simulink model "DCM_Controller_Implementation_Drive2"  (R2025a)
settings: Solver=ode5  StartTime=0.0  StopTime=t_end  FixedStep=dt  RelTol=1e-3
values from neighbouring files (symbols this model uses):
  a1 = -1.122    [Experiment_2_DCM_Parameter.m]
  a2 = 2.553    [Experiment_2_DCM_Parameter.m]
  a3 = -0.759    [Experiment_2_DCM_Parameter.m]
  b1 = 0.0876    [Experiment_2_DCM_Parameter.m]
  b2 = 0.1030    (= 0.103)    [Experiment_2_DCM_Parameter.m]
  b3 = 4.8586    [Experiment_2_DCM_Parameter.m]
  C_M = 0.96    [Experiment_2_DCM_Parameter.m]
  dt = 5e-6    (= 5e-06)    [Experiment_2_DCM_Parameter.m]
  dt_omega = 5e-4    (= 0.0005)    [Experiment_2_DCM_Parameter.m]
  EncoderLines = 4096    [Experiment_2_DCM_Parameter.m]
  I_AN = 1    [Experiment_2_DCM_Parameter.m]
  I_EN = 0.1    [Experiment_2_DCM_Parameter.m]
  K_i_i = V_r_I_A/T_n_I_A    (= 16.6666666667)    [Experiment_2_DCM_Parameter.m]
  K_i_omega = V_r_omega_m/T_n_omega_m    (= 4.70196759259)    [Experiment_2_DCM_Parameter.m]
  K_p_i = V_r_I_A    (= 0.283333333333)    [Experiment_2_DCM_Parameter.m]
  K_p_omega = V_r_omega_m    (= 0.112847222222)    [Experiment_2_DCM_Parameter.m]
  n_Igain = 0.075    [Experiment_2_DCM_Parameter.m]
  n_Imax = 0.15    [Experiment_2_DCM_Parameter.m]
  n_Imin = -n_Imax    (= -0.15)    [Experiment_2_DCM_Parameter.m]
  Omega_MN = N_N*pi/30    (= 209.439510239)    [Experiment_2_DCM_Parameter.m]
  Psi_EN = 1    [Experiment_2_DCM_Parameter.m]
  R_A = 22    [Experiment_2_DCM_Parameter.m]
  R_E = 2200    [Experiment_2_DCM_Parameter.m]
  T_A = L_A/R_A    (= 0.017)    [Experiment_2_DCM_Parameter.m]
  T_c = 1/1000    (= 0.001)    [Experiment_2_DCM_Parameter.m]
  T_CON = T_c    (= 0.001)    [Experiment_2_DCM_Parameter.m]
  Theta_M = 0.0013    [Experiment_2_DCM_Parameter.m]
  U_dc = 220    [Experiment_2_DCM_Parameter.m]
  U_EN = 220    [Experiment_2_DCM_Parameter.m]
  V_CON = 220    [Experiment_2_DCM_Parameter.m]
libraries: spsIGBTDiodeLib x4, simulink x3, spsGroundLib x1, spsDCVoltageSourceLib x1, spsVoltageMeasurementLib x1, sps_lib x1
settings Model: Creator=BinLi  LastModifiedBy=lucaslee
settings SolverCC: AlgebraicLoopSolver=TrustRegion
settings DataIOCC: LimitDataPoints=on  SaveFormat=Array  ReturnWorkspaceOutputs=off
settings OptimizationCC: BlockReduction=off  BooleanDataType=off  LifeSpan=inf
settings DebuggingCC: SaveWithParameterizedLinksMsg=none  UnderspecifiedInitializationDetection=Classic  MergeDetectMultiDrivingBlocksExec=none  SignalResolutionControl=TryResolveAllWithWarning  UnconnectedInputMsg=warning  UnconnectedOutputMsg=warning  UnconnectedLineMsg=warning  SFUnexpectedBacktrackingDiag=warning  SFNoUnconditionalDefaultTransitionDiag=warning  SFExecutionAtInitializationDiag=none  ArithmeticOperatorsInVariantConditions=warning
settings HardwareCC: ProdBitPerPointer=32.0  ProdBitPerSizeT=32.0  ProdBitPerPtrDiffT=32.0  ProdLargestAtomicFloat=None  ProdIntDivRoundTo=Undefined  ProdEndianess=Unspecified  ProdWordSize=32.0  ProdHWDeviceType=32-bit Generic  TargetUnknown=on
settings ModelReferenceCC: EnableRefExpFcnMdlSchedulingChecks=on  PropagateSignalLabelsOutOfModel=off
settings SFSimCC: SimUseLocalCustomCode=off  CustomCodeUndefinedFunction=UseInterfaceOnly
settings RTWCC: RTWUseLocalCustomCode=off  GPUComputeCapability=3.5
settings CodeAppCC: StateflowObjectComments=on
settings GRTTargetCC: TargetLangStandard=C89/C90 (ANSI)
settings ConfigComp: CovMetricSettings=dw  CovSaveCumulativeToWorkspaceVar=on  CovSaveSingleToWorkspaceVar=on  CovExternalEMLEnable=off  CovSFcnEnable=off

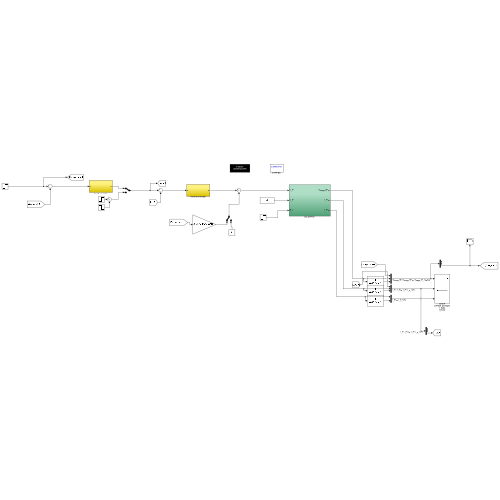
[thumbnail: Simulink's stored preview of the top-level diagram]
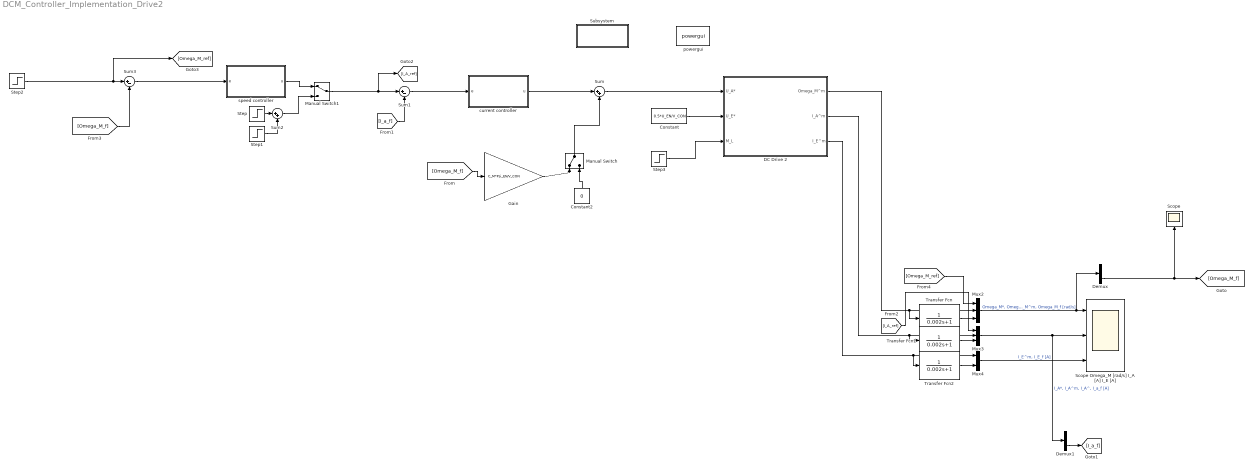
== system DCM_Controller_Implementation_Drive2 ==
  Constant : Constant  Value=0.5*U_EN/V_CON
  Constant2 : Constant  Value=0
  DC Drive 2 : Subsystem
  Demux : Demux  Outputs=3
  Demux1 : Demux  Outputs=3
  Gain : Gain  Gain=C_M*Psi_EN/V_CON
  Manual Switch : ManualSwitch
  Manual Switch1 : ManualSwitch
  Mux2 : Mux  Inputs=3
  Mux3 : Mux  Inputs=3
  Mux4 : Mux  Inputs=2
  Scope : Scope
      settings: ActiveDisplayYMinimum=-1  ActiveDisplayYMaximum=1
  Scope Omega_M [rad/s] I_A [A] I_E [A] : Scope  NumInputPorts=3
      settings: ActiveDisplayYMinimum=-32.249389430649124  ActiveDisplayYMaximum=259.56488911812932  DataLoggingSaveFormat=Array
  Step : Step  Time=0.5  After=I_AN/2  SampleTime=0
  Step1 : Step  After=-I_AN/2  SampleTime=0
  Step2 : Step  Time=0.5  After=1.1*Omega_MN  SampleTime=0
  Step3 : Step  After=0  SampleTime=0
  Subsystem : Subsystem
      settings: OpenFcn=Experiment_2_DCM_Parameter
      mask Display: disp('Initialize\n (doppelklicken)')
  Sum : Sum  Inputs=|++
  Sum1 : Sum  Inputs=|+-
  Sum2 : Sum  Inputs=|++
  Sum3 : Sum  Inputs=|+-
  Transfer Fcn : TransferFcn  Denominator=[0.002 1]
  Transfer Fcn1 : TransferFcn  Denominator=[0.002 1]
  Transfer Fcn2 : TransferFcn  Denominator=[0.002 1]
  current controller : Subsystem
  powergui : sps_lib/powergui  Priority=1  SimulationMode=Continuous  SampleTime=50e-6  frequency=60  Iterations=50  frequencyindice=0  Pbase=100e6  ErrMax=1e-4  UnitsV=kV  UnitsW=MW  buscounter=0  FunctionMessages=off  echomessages=off  EnableUseOfTLC=off  CurrentSourceSwitches=off  DisableSnubberDevices=off  DisableRonSwitches=off  DisableVfSwitches=off  DisplayEquations=off  AutomaticDiscreteSolvers=off  SolverType=Tustin/Backward Euler (TBE)  Interpol=off  ExternalGateDelay=off  methode=off  Ts=100  x0status=blocks  SPID=off  SwTol=0  HookPort=off  NonlinearTolerance=1e-4  nMaxIteration=100  ContinueOnMaxIteration=off  RestoreLinks=warning  ResistiveCurrentMeasurement=off  Frange=[0:2:500]  Ylog=off  Xlog=on  ShowGrid=off  save=off  variable=ZData  structure=0  ZoomFFT=off  StartTime=0.0  cycles=1  DisplayStyle=1  fundamental=60  FreqAxis=off  MaxFrequency=1000  frequencyindicesteady=1  RmsSteady=1  display=off
  speed controller : Subsystem
  wires:
  Mux2/1 -> Demux/1, Scope Omega_M [rad/s] I_A [A] I_E [A]/1  "Omega_M*, Omega_M^m, Omega_M_f [rad/s]"
  Mux3/1 -> Scope Omega_M [rad/s] I_A [A] I_E [A]/2, Demux1/1  "I_A*, I_A^m, I_A^, I_a_f [A]"
  Mux4/1 -> Scope Omega_M [rad/s] I_A [A] I_E [A]/3  "I_E^m, I_E_f [A]"
  DC Drive 2/2(I_A^m) -> Transfer Fcn1/1, Mux3/2
  DC Drive 2/3(I_E^m) -> Transfer Fcn2/1, Mux4/1
  DC Drive 2/1(Omega_M^m) -> Transfer Fcn/1, Mux2/2
  Transfer Fcn/1 -> Mux2/3
  Transfer Fcn2/1 -> Mux4/2
  Transfer Fcn1/1 -> Mux3/3
  Sum/1 -> DC Drive 2/1(U_A*)
  Demux/3 -> Scope/1, [Omega_M_f]
  [Omega_M_f] -> Gain/1
  current controller/1(u) -> Sum/1
  Sum1/1 -> current controller/1(e)
  [I_a_f] -> Sum1/2
  Demux1/3 -> [I_a_f]
  [I_A_ref] -> Mux3/1
  Constant/1 -> DC Drive 2/2(U_E*)
  Step/1 -> Sum2/1
  Step1/1 -> Sum2/2
  Step3/1 -> DC Drive 2/3(M_L)
  Manual Switch/1 -> Sum/2
  Gain/1 -> Manual Switch/1
  Constant2/1 -> Manual Switch/2
  Sum2/1 -> Manual Switch1/2
  speed controller/1(u) -> Manual Switch1/1
  Sum3/1 -> speed controller/1(e)
  [Omega_M_f] -> Sum3/2
  [Omega_M_ref] -> Mux2/1
  Step2/1 -> Sum3/1, [Omega_M_ref]
  Manual Switch1/1 -> [I_A_ref], Sum1/1

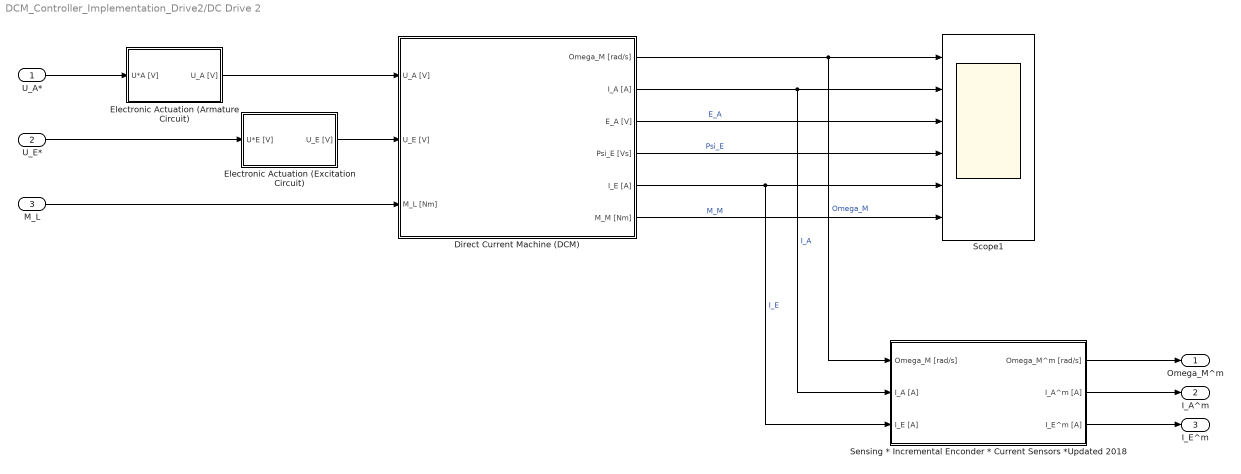
== system DCM_Controller_Implementation_Drive2/DC Drive 2 ==
  U_A* : Inport
  U_E* : Inport  Port=2
  M_L : Inport  Port=3
  Direct Current Machine (DCM) : Subsystem
  Electronic Actuation (Armature Circuit) : Subsystem
  Electronic Actuation (Excitation Circuit) : Subsystem
  Scope1 : Scope  NumInputPorts=6
      settings: DataLoggingSaveFormat=Array
  Sensing * Incremental Enconder * Current Sensors *Updated 2018 : Subsystem
  Omega_M^m : Outport
  I_A^m : Outport  Port=2
  I_E^m : Outport  Port=3
  wires:
  Electronic Actuation (Armature Circuit)/1(U_A [V]) -> Direct Current Machine (DCM)/1(U_A [V])
  Electronic Actuation (Excitation Circuit)/1(U_E [V]) -> Direct Current Machine (DCM)/2(U_E [V])
  U_E*/1 -> Electronic Actuation (Excitation Circuit)/1(U*E [V])
  M_L/1 -> Direct Current Machine (DCM)/3(M_L [Nm])
  U_A*/1 -> Electronic Actuation (Armature Circuit)/1(U*A [V])
  Direct Current Machine (DCM)/1(Omega_M [rad/s]) -> Sensing * Incremental Enconder * Current Sensors *Updated 2018/1(Omega_M [rad/s]), Scope1/1  "Omega_M"
  Direct Current Machine (DCM)/2(I_A [A]) -> Sensing * Incremental Enconder * Current Sensors *Updated 2018/2(I_A [A]), Scope1/2  "I_A"
  Direct Current Machine (DCM)/5(I_E [A]) -> Sensing * Incremental Enconder * Current Sensors *Updated 2018/3(I_E [A]), Scope1/5  "I_E"
  Direct Current Machine (DCM)/3(E_A [V]) -> Scope1/3  "E_A"
  Direct Current Machine (DCM)/4(Psi_E [Vs]) -> Scope1/4  "Psi_E"
  Direct Current Machine (DCM)/6(M_M [Nm]) -> Scope1/6  "M_M"
  Sensing * Incremental Enconder * Current Sensors *Updated 2018/1(Omega_M^m [rad/s]) -> Omega_M^m/1
  Sensing * Incremental Enconder * Current Sensors *Updated 2018/2(I_A^m [A]) -> I_A^m/1
  Sensing * Incremental Enconder * Current Sensors *Updated 2018/3(I_E^m [A]) -> I_E^m/1

== system DCM_Controller_Implementation_Drive2/Subsystem ==

== system DCM_Controller_Implementation_Drive2/current controller ==
  note: Create a PI-Controller with the Elements below.
  e : Inport
  Integrator : Integrator
  K_I : Gain  Gain=K_i_i
  K_P : Gain  Gain=K_p_i
  Sum : Sum  Inputs=|++
  u : Outport
  wires:
  e/1 -> K_I/1, K_P/1
  K_P/1 -> Sum/1
  K_I/1 -> Integrator/1
  Integrator/1 -> Sum/2
  Sum/1 -> u/1

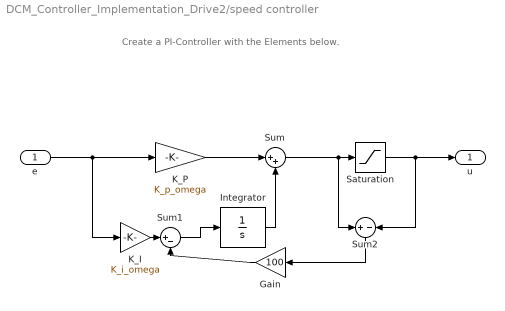
== system DCM_Controller_Implementation_Drive2/speed controller ==
  note: Create a PI-Controller with the Elements below.
  e : Inport
  Gain : Gain  Gain=100
  Integrator : Integrator
  K_I : Gain  Gain=K_i_omega
  K_P : Gain  Gain=K_p_omega
  Saturation : Saturate  UpperLimit=2  LowerLimit=-2
  Sum : Sum  Inputs=|++
  Sum1 : Sum  Inputs=|+-
  Sum2 : Sum  Inputs=+|-
  u : Outport
  wires:
  e/1 -> K_I/1, K_P/1
  K_P/1 -> Sum/1
  Sum/1 -> Sum2/1, Saturation/1
  Integrator/1 -> Sum/2
  Saturation/1 -> Sum2/2, u/1
  K_I/1 -> Sum1/1
  Sum1/1 -> Integrator/1
  Sum2/1 -> Gain/1
  Gain/1 -> Sum1/2

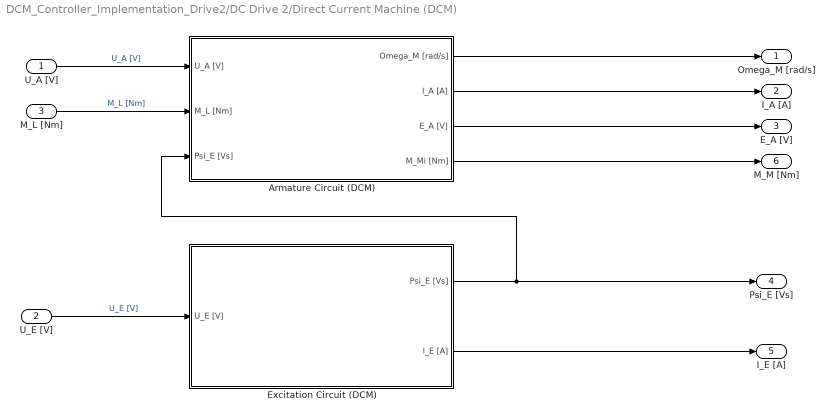
== system DCM_Controller_Implementation_Drive2/DC Drive 2/Direct Current Machine (DCM) ==
  U_A [V] : Inport
  U_E [V] : Inport  Port=2
  M_L [Nm] : Inport  Port=3
  Armature Circuit (DCM) : Subsystem
  Excitation Circuit (DCM) : Subsystem
  Omega_M [rad/s] : Outport  InitialOutput=0
  I_A [A] : Outport  Port=2  InitialOutput=0
  E_A [V] : Outport  Port=3  InitialOutput=0
  Psi_E [Vs] : Outport  Port=4  InitialOutput=0
  I_E [A] : Outport  Port=5  InitialOutput=0
  M_M [Nm] : Outport  Port=6  InitialOutput=0
  wires:
  Armature Circuit (DCM)/4(M_Mi [Nm]) -> M_M [Nm]/1
  Excitation Circuit (DCM)/2(I_E [A]) -> I_E [A]/1
  Armature Circuit (DCM)/3(E_A [V]) -> E_A [V]/1
  Armature Circuit (DCM)/2(I_A [A]) -> I_A [A]/1
  U_E [V]/1 -> Excitation Circuit (DCM)/1(U_E [V])  "U_E [V]"
  Armature Circuit (DCM)/1(Omega_M [rad/s]) -> Omega_M [rad/s]/1
  Excitation Circuit (DCM)/1(Psi_E [Vs]) -> Psi_E [Vs]/1, Armature Circuit (DCM)/3(Psi_E [Vs])
  M_L [Nm]/1 -> Armature Circuit (DCM)/2(M_L [Nm])  "M_L [Nm]"
  U_A [V]/1 -> Armature Circuit (DCM)/1(U_A [V])  "U_A [V]"

== system DCM_Controller_Implementation_Drive2/DC Drive 2/Electronic Actuation (Armature Circuit) ==
  U*A [V] : Inport
  Modulator : Subsystem
  Pulssteller : Subsystem
  U_A [V] : Outport
  wires:
  U*A [V]/1 -> Modulator/1(U_A*)
  Modulator/1(PWM_OUT) -> Pulssteller/1(PWM_IN)
  Pulssteller/1(u_A) -> U_A [V]/1

== system DCM_Controller_Implementation_Drive2/DC Drive 2/Electronic Actuation (Excitation Circuit) ==
  U*E [V] : Inport
  Dynamic Approximation of the 2-level-converter (Delay by T_CON) : TransportDelay  DelayTime=T_CON
  Gain : Gain  Gain=V_CON
  Saturation : Saturate  UpperLimit=U_dc  LowerLimit=-U_dc
  U_E [V] : Outport
  wires:
  Gain/1 -> Dynamic Approximation of the 2-level-converter (Delay by T_CON)/1
  U*E [V]/1 -> Gain/1  "U_E* [V]"
  Dynamic Approximation of the 2-level-converter (Delay by T_CON)/1 -> Saturation/1  "U_E [V]"
  Saturation/1 -> U_E [V]/1

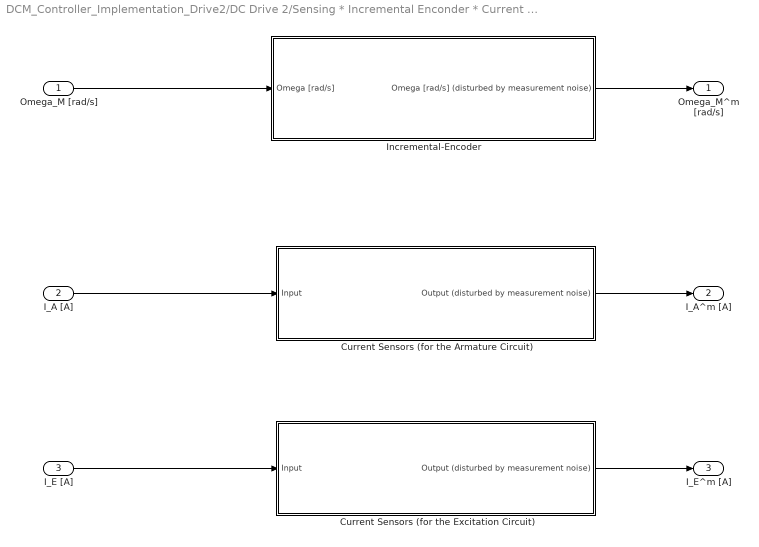
== system DCM_Controller_Implementation_Drive2/DC Drive 2/Sensing * Incremental Enconder * Current Sensors *Updated 2018 ==
  Omega_M [rad/s] : Inport
  I_A [A] : Inport  Port=2
  I_E [A] : Inport  Port=3
  Current Sensors (for the Armature Circuit) : Subsystem  mask(Noise Generator){Noise_Power=0.1*dt, h_Noise=dt, V_Noise=n_Igain, Max_Noise=n_Imax*I_AN, Min_Noise=n_Imin*I_AN}
      mask prompts: Noise_Power "Noise Power (default: 0.1*h)"; h_Noise "Noise Sampling Time (default: h)"; V_Noise "Noise Gain (Amplification)"; Max_Noise "Maximal Noise Amplitude (Saturation)"; Min_Noise "Minimal Noise Amplitude (Saturation)"
      mask help:
      | This block generates sensor noise (band limited white noise) at a noise sampling time h_Noise [s, default: h] and with a noise power Noise_Power [1, default: 0.1*h], to produce normally distributed bandlimited white noise with a maximal amplitude around 1.
      | The noise amplitude can be amplified with a noise gain V_Noise [1] and saturated with the maximal and minimal noise amplitude selection.
      | With the flag "ENABLE_NOISE" (constant) the noise output can be activated or set to zero.
      mask Display:
      | fprintf('Noise Power: %1.3f [1]\n Noise Sampling Time: %1.3f [s] \n Noise Gain: %g [1] \n Saturation: [%g,%g]'...
      |    ,Noise_Power, h_Noise, V_Noise, Min_Noise, Max_Noise);
      | port_label('input',1,'I [A]');
      | port_label('output',1,'I^m [A]');
  "Current Sensors (for the Excitation Circuit) " : Subsystem  mask(Noise Generator){Noise_Power=0.1*dt, h_Noise=dt, V_Noise=n_Igain, Max_Noise=n_Imax*I_EN, Min_Noise=n_Imin*I_EN}
      mask prompts: Noise_Power "Noise Power (default: 0.1*h)"; h_Noise "Noise Sampling Time (default: h)"; V_Noise "Noise Gain (Amplification)"; Max_Noise "Maximal Noise Amplitude (Saturation)"; Min_Noise "Minimal Noise Amplitude (Saturation)"
      mask help:
      | This block generates sensor noise (band limited white noise) at a noise sampling time h_Noise [s, default: h] and with a noise power Noise_Power [1, default: 0.1*h], to produce normally distributed bandlimited white noise with a maximal amplitude around 1.
      | The noise amplitude can be amplified with a noise gain V_Noise [1] and saturated with the maximal and minimal noise amplitude selection.
      | With the flag "ENABLE_NOISE" (constant) the noise output can be activated or set to zero.
      mask Display:
      | fprintf('Noise Power: %1.3f [1]\n Noise Sampling Time: %1.3f [s] \n Noise Gain: %g [1] \n Saturation: [%g,%g]'...
      |    ,Noise_Power, h_Noise, V_Noise, Min_Noise, Max_Noise);
      | port_label('input',1,'I [A]');
      | port_label('output',1,'I^m [A]');
  Incremental-Encoder : Subsystem  mask(Noise Generator){enc_lines=EncoderLines}
      mask prompts: enc_lines "Encoder Lines"
      mask help:
      | This block generates sensor noise (band limited white noise) at a noise sampling time h_Noise [s, default: h] and with a noise power Noise_Power [1, default: 0.1*h], to produce normally distributed bandlimited white noise with a maximal amplitude around 1.
      | The noise amplitude can be amplified with a noise gain V_Noise [1] and saturated with the maximal and minimal noise amplitude selection.
      | With the flag "ENABLE_NOISE" (constant) the noise output can be activated or set to zero.
      mask Display:
      | fprintf('Encoder Lines %g [1]',enc_lines);
      | port_label('input',1,'Omega [rad/s]');
      | port_label('output',1,'Omega^m [rad/s]');
  Omega_M^m [rad/s] : Outport  InitialOutput=0
  I_A^m [A] : Outport  Port=2  InitialOutput=0
  I_E^m [A] : Outport  Port=3  InitialOutput=0
  wires:
  Omega_M [rad/s]/1 -> Incremental-Encoder/1(Omega [rad/s])
  I_A [A]/1 -> Current Sensors (for the Armature Circuit)/1(Input)
  I_E [A]/1 -> "Current Sensors (for the Excitation Circuit) "/1(Input)
  "Current Sensors (for the Excitation Circuit) "/1(Output (disturbed by measurement noise)) -> I_E^m [A]/1
  Current Sensors (for the Armature Circuit)/1(Output (disturbed by measurement noise)) -> I_A^m [A]/1
  Incremental-Encoder/1(Omega [rad/s] (disturbed by measurement noise)) -> Omega_M^m [rad/s]/1

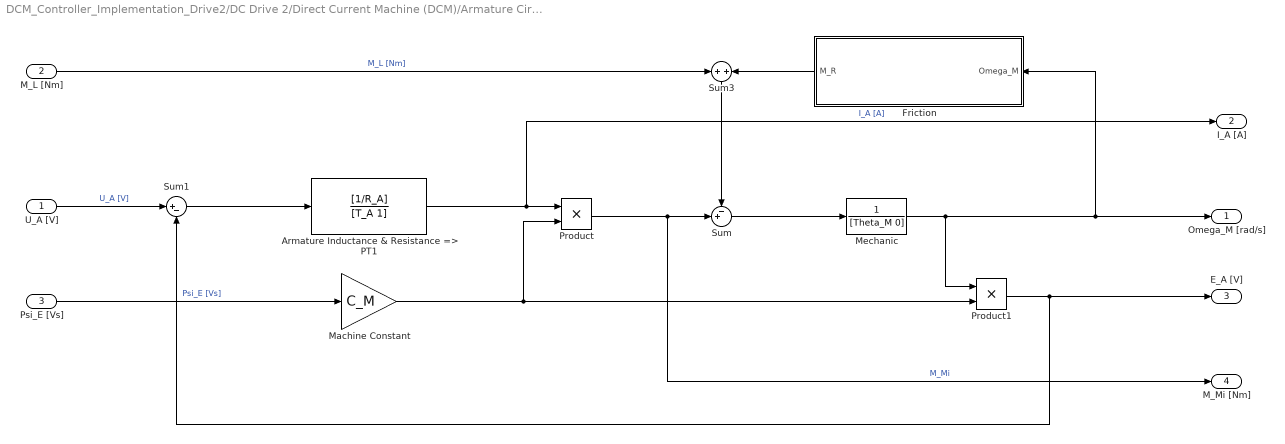
== system DCM_Controller_Implementation_Drive2/DC Drive 2/Direct Current Machine (DCM)/Armature Circuit (DCM) ==
  U_A [V] : Inport
  M_L [Nm] : Inport  Port=2
  Psi_E [Vs] : Inport  Port=3
  Armature Inductance & Resistance => PT1 : TransferFcn  Numerator=[1/R_A]  Denominator=[T_A 1]
  Friction : Subsystem
  Machine Constant : Gain  Gain=C_M
  Mechanic : TransferFcn  Denominator=[Theta_M 0]
  Product : Product  RndMeth=Zero
  Product1 : Product  RndMeth=Zero
  Sum : Sum  Inputs=-+|
  Sum1 : Sum  Inputs=|+-
  Sum3 : Sum  Inputs=+|+
  Omega_M [rad/s] : Outport  InitialOutput=0
  I_A [A] : Outport  Port=2  InitialOutput=0
  E_A [V] : Outport  Port=3  InitialOutput=0
  M_Mi [Nm] : Outport  Port=4  InitialOutput=0
  wires:
  Psi_E [Vs]/1 -> Machine Constant/1  "Psi_E [Vs]"
  Armature Inductance & Resistance => PT1/1 -> Product/1, I_A [A]/1  "I_A [A]"
  M_L [Nm]/1 -> Sum3/1  "M_L [Nm]"
  Product/1 -> M_Mi [Nm]/1, Sum/2  "M_Mi"
  Machine Constant/1 -> Product1/2, Product/2
  U_A [V]/1 -> Sum1/1  "U_A [V]"
  Sum1/1 -> Armature Inductance & Resistance => PT1/1
  Sum/1 -> Mechanic/1
  Mechanic/1 -> Friction/1(Omega_M), Omega_M [rad/s]/1, Product1/1
  Product1/1 -> Sum1/2, E_A [V]/1
  Sum3/1 -> Sum/1
  Friction/1(M_R) -> Sum3/2

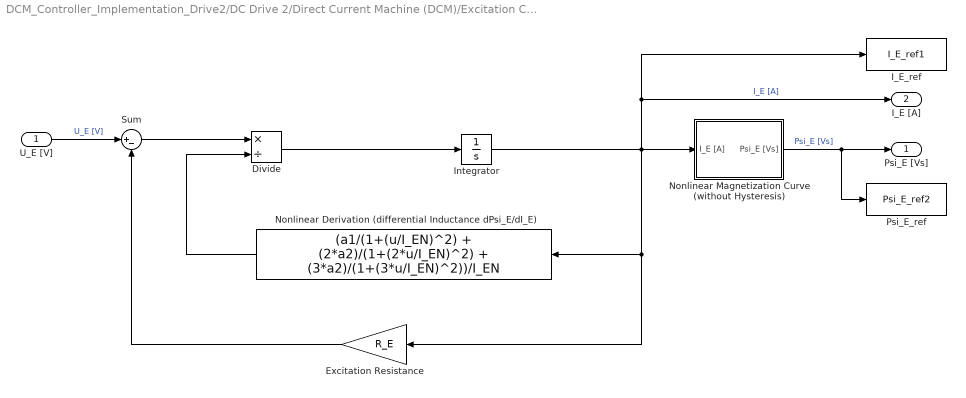
== system DCM_Controller_Implementation_Drive2/DC Drive 2/Direct Current Machine (DCM)/Excitation Circuit (DCM) ==
  U_E [V] : Inport
  Divide : Product  Inputs=*/
  Excitation Resistance : Gain  Gain=R_E
  I_E_ref : ToWorkspace  VariableName=I_E_ref1  SampleTime=-1
  Integrator : Integrator
  Nonlinear Derivation (differential Inductance dPsi_E/dI_E) : Fcn  Expr=(a1/(1+(u/I_EN)^2) + (2*a2)/(1+(2*u/I_EN)^2) + (3*a2)/(1+(3*u/I_EN)^2))/I_EN
  Nonlinear Magnetization Curve (without Hysteresis) : Subsystem
      mask Display:
      | plot([-5:0.1:5], 2/pi*atan([-5:0.1:5]./1.5) + 0.05.*[-5:0.1:5]);
      | plot([0 0],[-1.25 1.25]);
      | plot([-5 5],[0 0]);
  Psi_E_ref : ToWorkspace  VariableName=Psi_E_ref2  SampleTime=-1
  Sum : Sum  Inputs=|+-  InputSameDT=on  SaturateOnIntegerOverflow=on  OutDataTypeStr=Inherit: Same as first input
  Psi_E [Vs] : Outport  InitialOutput=0
  I_E [A] : Outport  Port=2  InitialOutput=0
  wires:
  Nonlinear Magnetization Curve (without Hysteresis)/1(Psi_E [Vs]) -> Psi_E_ref/1, Psi_E [Vs]/1  "Psi_E [Vs]"
  U_E [V]/1 -> Sum/1  "U_E [V]"
  Excitation Resistance/1 -> Sum/2
  Sum/1 -> Divide/1
  Nonlinear Derivation (differential Inductance dPsi_E/dI_E)/1 -> Divide/2
  Integrator/1 -> I_E_ref/1, I_E [A]/1, Nonlinear Magnetization Curve (without Hysteresis)/1(I_E [A]), Excitation Resistance/1, Nonlinear Derivation (differential Inductance dPsi_E/dI_E)/1  "I_E [A]"
  Divide/1 -> Integrator/1

== system DCM_Controller_Implementation_Drive2/DC Drive 2/Electronic Actuation (Armature Circuit)/Modulator ==
  U_A* : Inport
  Relay : Relay  OnSwitchValue=1e-4  OffSwitchValue=-1e-4
  Scope : Scope
      settings: DataLoggingSaveFormat=Array
  Sum1 : Sum  Inputs=|+-
  u_d : simulink/Sources/Repeating Sequence  rep_seq_t=[0 T_c/2 T_c]  rep_seq_y=[1 -1 1]
  PWM_OUT : Outport
  wires:
  u_d/1 -> Sum1/2
  Sum1/1 -> Relay/1
  Relay/1 -> Scope/1, PWM_OUT/1
  U_A*/1 -> Sum1/1

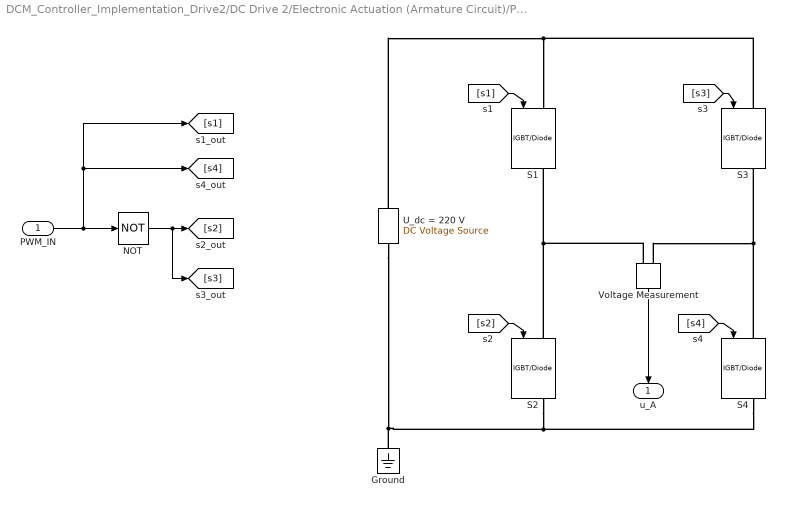
== system DCM_Controller_Implementation_Drive2/DC Drive 2/Electronic Actuation (Armature Circuit)/Pulssteller ==
  PWM_IN : Inport
  Ground : spsGroundLib/Ground  LConnTagsString=a
  NOT : Logic  Operator=NOT  AllPortsSameDT=off  OutDataTypeStr=boolean
  S{1..4} (4 alike) : spsIGBTDiodeLib/IGBT//Diode  Ron=1e-3  Rs=1e5  Cs=inf  Measurements=on
  U_dc = 220 V : spsDCVoltageSourceLib/DC Voltage Source  Amplitude=U_dc  Measurements=None
  Voltage Measurement : spsVoltageMeasurementLib/Voltage Measurement  Tag=PoWeRsYsTeMmEaSuReMeNt  PhasorSimulation=off  OutputType=Complex  PSBequivalent=0
  u_A : Outport
  wires:
  [s2] -> S2/1
  NOT/1 -> [s3], [s2]
  PWM_IN/1 -> [s4], [s1], NOT/1
  [s1] -> S1/1
  [s3] -> S3/1
  [s4] -> S4/1
  Voltage Measurement/1 -> u_A/1
  connections:
  S4/LConn1 -- Voltage Measurement/LConn2 -- S3/RConn1
  S2/LConn1 -- S1/RConn1 -- Voltage Measurement/LConn1
  S3/LConn1 -- U_dc = 220 V/RConn1 -- S1/LConn1
  S2/RConn1 -- U_dc = 220 V/LConn1 -- Ground/LConn1 -- S4/RConn1

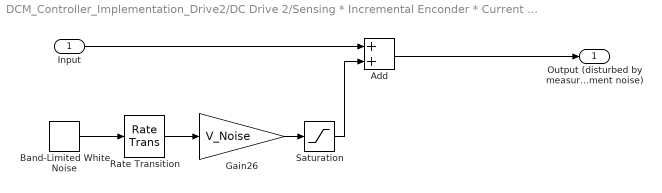
== system DCM_Controller_Implementation_Drive2/DC Drive 2/Sensing * Incremental Enconder * Current Sensors *Updated 2018/Current Sensors (for the Armature Circuit) ==
  Input : Inport
  Add : Sum
  Band-Limited White Noise : simulink/Sources/Band-Limited White Noise  Cov=[Noise_Power]  Ts=h_Noise  seed=[23341]
  Gain26 : Gain  Gain=V_Noise
  Rate Transition : RateTransition  OutPortSampleTime=h_Noise
  Saturation : Saturate  UpperLimit=Max_Noise  LowerLimit=Min_Noise
  Output (disturbed by measurement noise) : Outport
  wires:
  Saturation/1 -> Add/2
  Input/1 -> Add/1
  Rate Transition/1 -> Gain26/1
  Gain26/1 -> Saturation/1
  Band-Limited White Noise/1 -> Rate Transition/1
  Add/1 -> Output (disturbed by measurement noise)/1

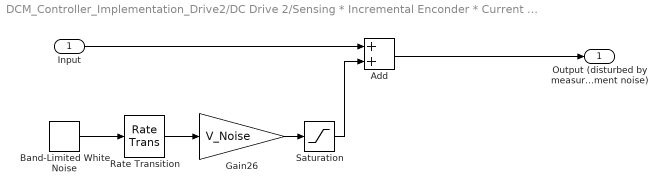
== system DCM_Controller_Implementation_Drive2/DC Drive 2/Sensing * Incremental Enconder * Current Sensors *Updated 2018/Current Sensors (for the Excitation Circuit)  ==
  Input : Inport
  Add : Sum
  Band-Limited White Noise : simulink/Sources/Band-Limited White Noise  Cov=[Noise_Power]  Ts=h_Noise  seed=[23341]
  Gain26 : Gain  Gain=V_Noise
  Rate Transition : RateTransition  OutPortSampleTime=h_Noise
  Saturation : Saturate  UpperLimit=Max_Noise  LowerLimit=Min_Noise
  Output (disturbed by measurement noise) : Outport
  wires:
  Band-Limited White Noise/1 -> Rate Transition/1
  Gain26/1 -> Saturation/1
  Rate Transition/1 -> Gain26/1
  Input/1 -> Add/1
  Saturation/1 -> Add/2
  Add/1 -> Output (disturbed by measurement noise)/1

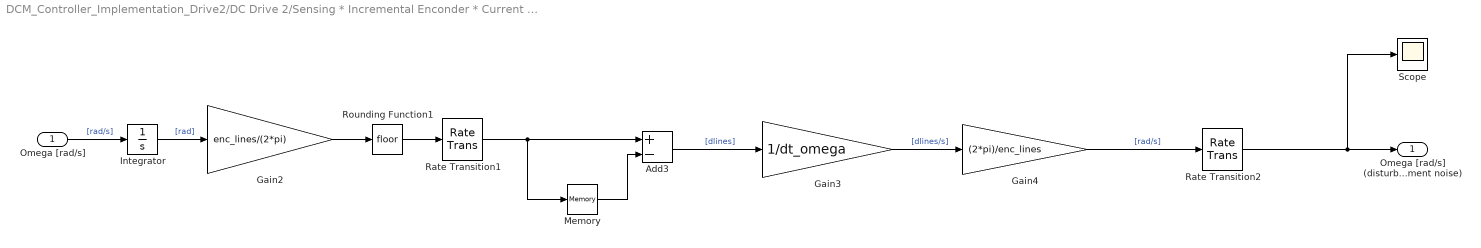
== system DCM_Controller_Implementation_Drive2/DC Drive 2/Sensing * Incremental Enconder * Current Sensors *Updated 2018/Incremental-Encoder ==
  Omega [rad/s] : Inport
  Add3 : Sum  Inputs=+-
  Gain2 : Gain  Gain=enc_lines/(2*pi)
  Gain3 : Gain  Gain=1/dt_omega
  Gain4 : Gain  Gain=(2*pi)/enc_lines
  Integrator : Integrator
  Memory : Memory  InheritSampleTime=on
  Rate Transition1 : RateTransition  OutPortSampleTime=dt_omega
  Rate Transition2 : RateTransition  OutPortSampleTime=dt
  Rounding Function1 : Rounding
  Scope : Scope
      settings: ActiveDisplayYMinimum=0  ActiveDisplayYMaximum=250  DataLoggingVariableName=ScopeData2
  Omega [rad/s] (disturbed by measurement noise) : Outport
  wires:
  Integrator/1 -> Gain2/1  "[rad]"
  Gain2/1 -> Rounding Function1/1
  Memory/1 -> Add3/2
  Add3/1 -> Gain3/1  "[dlines]"
  Gain3/1 -> Gain4/1  "[dlines/s]"
  Gain4/1 -> Rate Transition2/1  "[rad/s]"
  Rounding Function1/1 -> Rate Transition1/1
  Omega [rad/s]/1 -> Integrator/1  "[rad/s]"
  Rate Transition1/1 -> Memory/1, Add3/1
  Rate Transition2/1 -> Omega [rad/s] (disturbed by measurement noise)/1, Scope/1

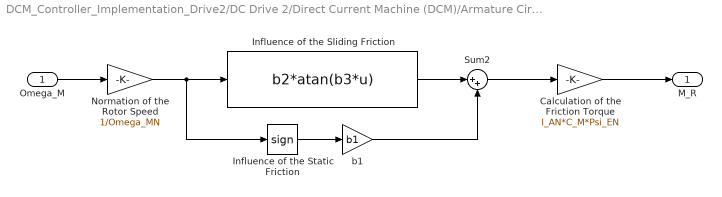
== system DCM_Controller_Implementation_Drive2/DC Drive 2/Direct Current Machine (DCM)/Armature Circuit (DCM)/Friction ==
  Omega_M : Inport
  Calculation of the Friction Torque : Gain  Gain=I_AN*C_M*Psi_EN
  Influence of the Static Friction : Signum
  "Influence of the Sliding Friction " : Fcn  Expr=b2*atan(b3*u)
  Normation of the Rotor Speed : Gain  Gain=1/Omega_MN
  Sum2 : Sum  Inputs=|++
  b1 : Gain  Gain=b1
  M_R : Outport
  wires:
  b1/1 -> Sum2/2
  "Influence of the Sliding Friction "/1 -> Sum2/1
  Influence of the Static Friction/1 -> b1/1
  Omega_M/1 -> Normation of the Rotor Speed/1
  Sum2/1 -> Calculation of the Friction Torque/1
  Calculation of the Friction Torque/1 -> M_R/1
  Normation of the Rotor Speed/1 -> Influence of the Static Friction/1, "Influence of the Sliding Friction "/1

== system DCM_Controller_Implementation_Drive2/DC Drive 2/Direct Current Machine (DCM)/Excitation Circuit (DCM)/Nonlinear Magnetization Curve (without Hysteresis) ==
  I_E [A] : Inport
  Nichtlineare Magnetisierungskennlinie (ohne Hysterese) : Fcn  Expr=(a1*atan(u/I_EN) + a2*atan(2*u/I_EN) + a3*atan(3*u/I_EN))
  Psi_E [Vs] : Outport
  wires:
  I_E [A]/1 -> Nichtlineare Magnetisierungskennlinie (ohne Hysterese)/1
  Nichtlineare Magnetisierungskennlinie (ohne Hysterese)/1 -> Psi_E [Vs]/1
